simulink model "stereo_ibvs_core"  (R2025b)
settings: Solver=FixedStepDiscrete  StartTime=0.0  StopTime=inf  FixedStep=cfg.Ts  RelTol=1e-3
InitFcn:
  | modelFile__ = get_param(bdroot,'FileName'); modelDir__ = fileparts(modelFile__); config1__ = fullfile(modelDir__,'stereo_ibvs_config.m'); config2__ = fullfile(fileparts(modelDir__),'config','stereo_ibvs_config.m'); if isfile(config1__), run(config1__); elseif isfile(config2__), run(config2__); else, error('StereoIBVS:ConfigNotFound','找不到stereo_ibvs_config.m。'); end; clear modelFile__ modelDir__ config1__ config2__;
undefined symbols (not defined in the file or in its folder): cfg
libraries: robotmaniplib x2
settings Model: Creator=harry  LastModifiedBy=hlc

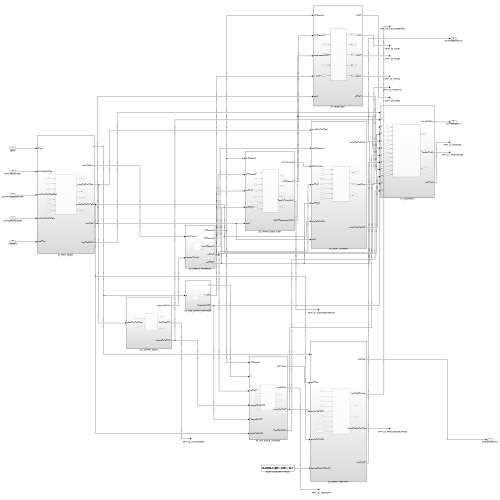
[thumbnail: Simulink's stored preview of the top-level diagram]
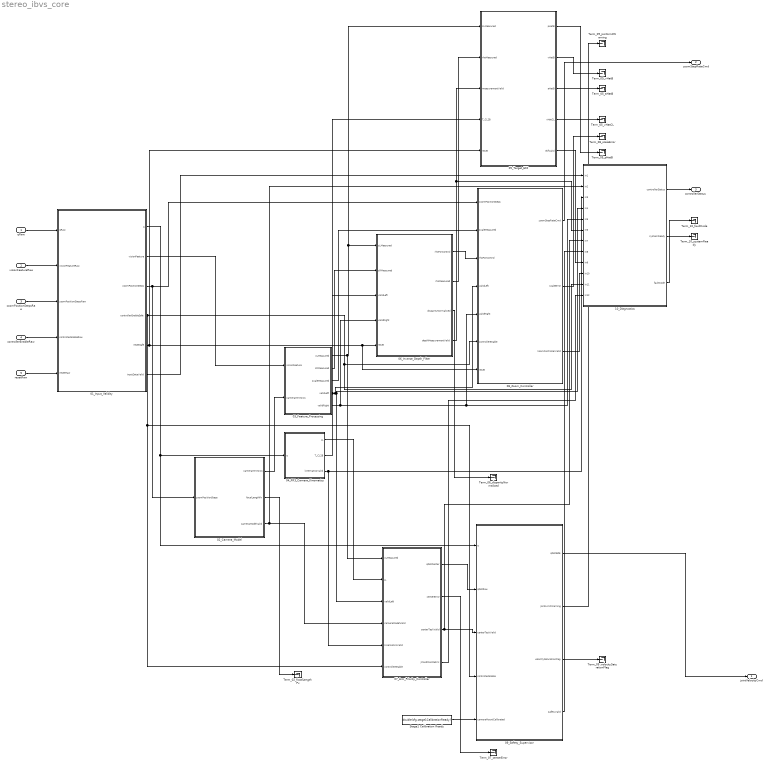
== system stereo_ibvs_core ==
  qRaw : Inport  OutDataTypeStr=double  PortDimensions=[7 1]
  visionFeatureRaw : Inport  Port=2  PortDimensions=[8 1]
  zoomPositionStepsRaw : Inport  Port=3  PortDimensions=[2 1]
  controllerEnableRaw : Inport  Port=4  OutDataTypeStr=double  PortDimensions=1
  resetRaw : Inport  Port=5  OutDataTypeStr=double  PortDimensions=1
  01_Input_Validity : Subsystem
  02_Camera_Model : Subsystem
  03_Feature_Processing : Subsystem  Description=将像素坐标转换为左右相机归一化坐标，并检查输入有效性。
  04_FR3_Camera_Kinematics : Subsystem
  05_Target_EKF : Subsystem
  06_Inverse_Depth_Filter : Subsystem
  07_Arm_Priority_Controller : Subsystem
  08_Zoom_Controller : Subsystem
  09_Safety_Supervisor : Subsystem
  10_Diagnostics : Subsystem
  Stage1 Calibration Ready : Constant  Value=double(cfg.stage1CalibrationReady)  SampleTime=-1
  Term_02_focalLengthPx : Terminator
  Term_05_aHatB : Terminator
  Term_05_pHatB : Terminator
  Term_05_vHatB : Terminator
  Term_05_vHatCL : Terminator
  Term_06_disparityNormalized : Terminator
  Term_07_centerError : Terminator
  Term_08_scaleError : Terminator
  Term_09_jointLimitWarning : Terminator
  Term_09_velocitySaturationFlag : Terminator
  Term_10_faultCode : Terminator
  Term_10_systemReady : Terminator
  jointVelocityCmd : Outport  PortDimensions=[7 1]
  zoomStepRateCmd : Outport  Port=2  PortDimensions=[2 1]
  controllerStatus : Outport  Port=3  PortDimensions=[12 1]
  wires:
  10_Diagnostics/3(faultCode) -> Term_10_faultCode/1
  10_Diagnostics/1(controllerStatus) -> controllerStatus/1
  09_Safety_Supervisor/4(safetyValid) -> 10_Diagnostics/8(In8)
  09_Safety_Supervisor/1(qDotSafe) -> jointVelocityCmd/1
  08_Zoom_Controller/2(scaleError) -> Term_08_scaleError/1
  05_Target_EKF/3(aHatB) -> Term_05_aHatB/1
  Stage1 Calibration Ready/1 -> 09_Safety_Supervisor/5(cameraMountCalibrated)
  08_Zoom_Controller/3(zoomControllerValid) -> 10_Diagnostics/10(In10)
  07_Arm_Priority_Controller/4(jConditionMetric) -> 10_Diagnostics/12(In12)
  01_Input_Validity/6(inputDataValid) -> 10_Diagnostics/1(In1)
  01_Input_Validity/5(resetSafe) -> 06_Inverse_Depth_Filter/5(reset), 08_Zoom_Controller/7(reset), 05_Target_EKF/5(reset)
  01_Input_Validity/2(visionFeature) -> 03_Feature_Processing/1(visionFeature)
  01_Input_Validity/1(q) -> 09_Safety_Supervisor/1(q), 04_FR3_Camera_Kinematics/1(q)
  02_Camera_Model/1(cameraIntrinsics) -> 03_Feature_Processing/2(cameraIntrinsics)
  02_Camera_Model/2(focalLengthPx) -> Term_02_focalLengthPx/1
  08_Zoom_Controller/1(zoomStepRateCmd) -> zoomStepRateCmd/1
  03_Feature_Processing/3(scaleMeasured) -> 08_Zoom_Controller/2(scaleMeasured)
  05_Target_EKF/4(vHatCL) -> Term_05_vHatCL/1
  resetRaw/1 -> 01_Input_Validity/5(resetRaw)
  controllerEnableRaw/1 -> 01_Input_Validity/4(controllerEnableRaw)
  07_Arm_Priority_Controller/1(qDotCenter) -> 09_Safety_Supervisor/2(qDotRaw)
  09_Safety_Supervisor/2(jointLimitWarning) -> Term_09_jointLimitWarning/1
  05_Target_EKF/5(ekfValid) -> 10_Diagnostics/9(In9)
  05_Target_EKF/1(pHatB) -> Term_05_pHatB/1
  zoomPositionStepsRaw/1 -> 01_Input_Validity/3(zoomPositionStepsRaw)
  visionFeatureRaw/1 -> 01_Input_Validity/2(visionFeatureRaw)
  06_Inverse_Depth_Filter/4(depthMeasurementValid) -> 05_Target_EKF/3(measurementValid), 10_Diagnostics/6(In6)
  01_Input_Validity/4(controllerEnableSafe) -> 09_Safety_Supervisor/4(controllerEnable), 07_Arm_Priority_Controller/6(controllerEnable), 08_Zoom_Controller/6(controllerEnable), 10_Diagnostics/11(In11)
  qRaw/1 -> 01_Input_Validity/1(qRaw)
  03_Feature_Processing/1(cLMeasured) -> 06_Inverse_Depth_Filter/1(cLMeasured), 05_Target_EKF/1(cLMeasured), 07_Arm_Priority_Controller/1(cLMeasured)
  03_Feature_Processing/4(validLeft) -> 07_Arm_Priority_Controller/3(validLeft), 10_Diagnostics/4(In4), 08_Zoom_Controller/4(validLeft), 06_Inverse_Depth_Filter/3(validLeft)
  03_Feature_Processing/5(validRight) -> 08_Zoom_Controller/5(validRight), 10_Diagnostics/5(In5), 06_Inverse_Depth_Filter/4(validRight)
  10_Diagnostics/2(systemReady) -> Term_10_systemReady/1
  02_Camera_Model/3(cameraModelValid) -> 10_Diagnostics/2(In2), 07_Arm_Priority_Controller/4(cameraModelValid)
  04_FR3_Camera_Kinematics/3(kinematicsValid) -> 07_Arm_Priority_Controller/5(kinematicsValid), 10_Diagnostics/3(In3)
  05_Target_EKF/2(vHatB) -> Term_05_vHatB/1
  07_Arm_Priority_Controller/3(centerTaskValid) -> 09_Safety_Supervisor/3(centerTaskValid), 10_Diagnostics/7(In7)
  09_Safety_Supervisor/3(velocitySaturationFlag) -> Term_09_velocitySaturationFlag/1
  04_FR3_Camera_Kinematics/2(T_CL2B) -> 05_Target_EKF/4(T_CL2B)
  03_Feature_Processing/2(cRMeasured) -> 06_Inverse_Depth_Filter/2(cRMeasured)
  06_Inverse_Depth_Filter/2(rhoMeasured) -> 05_Target_EKF/2(rhoMeasured)
  01_Input_Validity/3(zoomPositionSteps) -> 02_Camera_Model/1(zoomPositionSteps), 08_Zoom_Controller/1(zoomPositionSteps)
  07_Arm_Priority_Controller/2(centerError) -> Term_07_centerError/1
  06_Inverse_Depth_Filter/1(rhoForControl) -> 08_Zoom_Controller/3(rhoForControl)
  04_FR3_Camera_Kinematics/1(JL) -> 07_Arm_Priority_Controller/2(JL)
  06_Inverse_Depth_Filter/3(disparityNormalized) -> Term_06_disparityNormalized/1

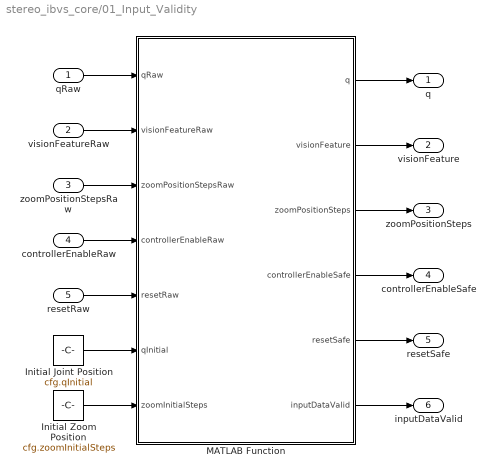
== system stereo_ibvs_core/01_Input_Validity ==
  qRaw : Inport  PortDimensions=[7 1]
  visionFeatureRaw : Inport  Port=2  PortDimensions=[8 1]
  zoomPositionStepsRaw : Inport  Port=3  PortDimensions=[2 1]
  controllerEnableRaw : Inport  Port=4  PortDimensions=1
  resetRaw : Inport  Port=5  PortDimensions=1
  Initial Joint Position : Constant  Value=cfg.qInitial  VectorParams1D=off
  Initial Zoom Position : Constant  Value=cfg.zoomInitialSteps  VectorParams1D=off
  MATLAB Function : MATLAB Function  TreatAsAtomicUnit=on
  q : Outport  PortDimensions=[7 1]
  visionFeature : Outport  Port=2  PortDimensions=[8 1]
  zoomPositionSteps : Outport  Port=3  PortDimensions=[2 1]
  controllerEnableSafe : Outport  Port=4  PortDimensions=1
  resetSafe : Outport  Port=5  PortDimensions=1
  inputDataValid : Outport  Port=6  PortDimensions=1
  wires:
  MATLAB Function/1(q) -> q/1
  MATLAB Function/2(visionFeature) -> visionFeature/1
  MATLAB Function/3(zoomPositionSteps) -> zoomPositionSteps/1
  MATLAB Function/4(controllerEnableSafe) -> controllerEnableSafe/1
  MATLAB Function/5(resetSafe) -> resetSafe/1
  MATLAB Function/6(inputDataValid) -> inputDataValid/1
  qRaw/1 -> MATLAB Function/1(qRaw)
  visionFeatureRaw/1 -> MATLAB Function/2(visionFeatureRaw)
  zoomPositionStepsRaw/1 -> MATLAB Function/3(zoomPositionStepsRaw)
  controllerEnableRaw/1 -> MATLAB Function/4(controllerEnableRaw)
  resetRaw/1 -> MATLAB Function/5(resetRaw)
  Initial Joint Position/1 -> MATLAB Function/6(qInitial)
  Initial Zoom Position/1 -> MATLAB Function/7(zoomInitialSteps)

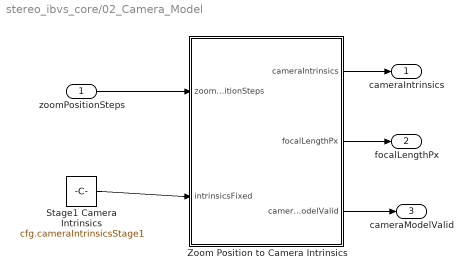
== system stereo_ibvs_core/02_Camera_Model ==
  zoomPositionSteps : Inport  PortDimensions=[2 1]
  Stage1 Camera Intrinsics : Constant  Value=cfg.cameraIntrinsicsStage1  VectorParams1D=off
  Zoom Position to Camera Intrinsics : MATLAB Function  TreatAsAtomicUnit=on
  cameraIntrinsics : Outport  PortDimensions=[8 1]
  focalLengthPx : Outport  Port=2  PortDimensions=[2 1]
  cameraModelValid : Outport  Port=3  PortDimensions=1
  wires:
  zoomPositionSteps/1 -> Zoom Position to Camera Intrinsics/1(zoomPositionSteps)
  Stage1 Camera Intrinsics/1 -> Zoom Position to Camera Intrinsics/2(intrinsicsFixed)
  Zoom Position to Camera Intrinsics/3(cameraModelValid) -> cameraModelValid/1
  Zoom Position to Camera Intrinsics/2(focalLengthPx) -> focalLengthPx/1
  Zoom Position to Camera Intrinsics/1(cameraIntrinsics) -> cameraIntrinsics/1

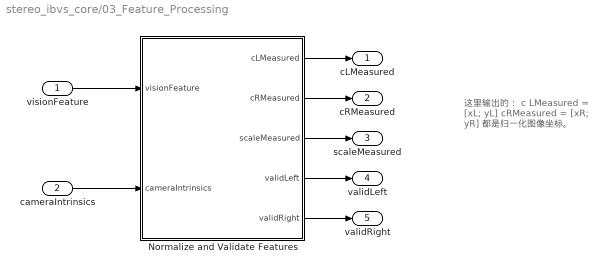
== system stereo_ibvs_core/03_Feature_Processing ==
  note: 这里输出的：
      | c LMeasured = [xL; yL]
      | cRMeasured = [xR; yR]
      | 都是归一化图像坐标。
  visionFeature : Inport  PortDimensions=[8 1]
  cameraIntrinsics : Inport  Description=|  Port=2  PortDimensions=[8 1]
      | 顺序固定为：
      | [fxL; fyL; cxL; cyL; fxR; fyR; cxR; cyR]
  Normalize and Validate Features : MATLAB Function  TreatAsAtomicUnit=on
  cLMeasured : Outport  PortDimensions=[2 1]
  cRMeasured : Outport  Port=2  PortDimensions=[2 1]
  scaleMeasured : Outport  Port=3  PortDimensions=[2 1]
  validLeft : Outport  Port=4  PortDimensions=1
  validRight : Outport  Port=5  PortDimensions=1
  wires:
  cameraIntrinsics/1 -> Normalize and Validate Features/2(cameraIntrinsics)
  visionFeature/1 -> Normalize and Validate Features/1(visionFeature)
  Normalize and Validate Features/2(cRMeasured) -> cRMeasured/1
  Normalize and Validate Features/4(validLeft) -> validLeft/1
  Normalize and Validate Features/5(validRight) -> validRight/1
  Normalize and Validate Features/3(scaleMeasured) -> scaleMeasured/1
  Normalize and Validate Features/1(cLMeasured) -> cLMeasured/1

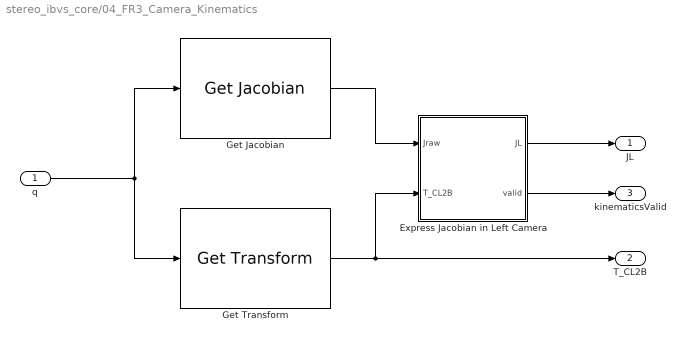
== system stereo_ibvs_core/04_FR3_Camera_Kinematics ==
  q : Inport  PortDimensions=[7 1]
  Express Jacobian in Left Camera : MATLAB Function  TreatAsAtomicUnit=on
  Get Jacobian : robotmaniplib/Get Jacobian  Description=关节速度如何产生左相机光心的运动速度。该速度默认在 base 坐标系表达  RigidBodyTree=cfg.robot  EndEffector=left_camera_optical  SimulateUsing=Interpreted execution
  Get Transform : robotmaniplib/Get Transform  Description=它把左相机坐标系(source)中的点转换到 base 坐标系(target)  RigidBodyTree=cfg.robot  SourceBody=left_camera_optical  TargetBody=base  SimulateUsing=Interpreted execution
  JL : Outport  PortDimensions=[6 7]
  T_CL2B : Outport  Port=2  PortDimensions=[4 4]
  kinematicsValid : Outport  Port=3  PortDimensions=1
  wires:
  q/1 -> Get Jacobian/1, Get Transform/1
  Get Jacobian/1 -> Express Jacobian in Left Camera/1(Jraw)
  Get Transform/1 -> T_CL2B/1, Express Jacobian in Left Camera/2(T_CL2B)
  Express Jacobian in Left Camera/1(JL) -> JL/1
  Express Jacobian in Left Camera/2(valid) -> kinematicsValid/1

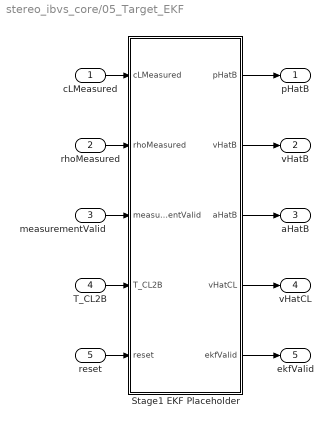
== system stereo_ibvs_core/05_Target_EKF ==
  cLMeasured : Inport  PortDimensions=[2 1]
  rhoMeasured : Inport  Port=2  PortDimensions=1
  measurementValid : Inport  Port=3  PortDimensions=1
  T_CL2B : Inport  Port=4  PortDimensions=[4 4]
  reset : Inport  Port=5  PortDimensions=1
  Stage1 EKF Placeholder : MATLAB Function  TreatAsAtomicUnit=on
  pHatB : Outport  PortDimensions=[3 1]
  vHatB : Outport  Port=2  PortDimensions=[3 1]
  aHatB : Outport  Port=3  PortDimensions=[3 1]
  vHatCL : Outport  Port=4  PortDimensions=[3 1]
  ekfValid : Outport  Port=5  PortDimensions=1
  wires:
  cLMeasured/1 -> Stage1 EKF Placeholder/1(cLMeasured)
  rhoMeasured/1 -> Stage1 EKF Placeholder/2(rhoMeasured)
  measurementValid/1 -> Stage1 EKF Placeholder/3(measurementValid)
  T_CL2B/1 -> Stage1 EKF Placeholder/4(T_CL2B)
  reset/1 -> Stage1 EKF Placeholder/5(reset)
  Stage1 EKF Placeholder/1(pHatB) -> pHatB/1
  Stage1 EKF Placeholder/2(vHatB) -> vHatB/1
  Stage1 EKF Placeholder/3(aHatB) -> aHatB/1
  Stage1 EKF Placeholder/4(vHatCL) -> vHatCL/1
  Stage1 EKF Placeholder/5(ekfValid) -> ekfValid/1

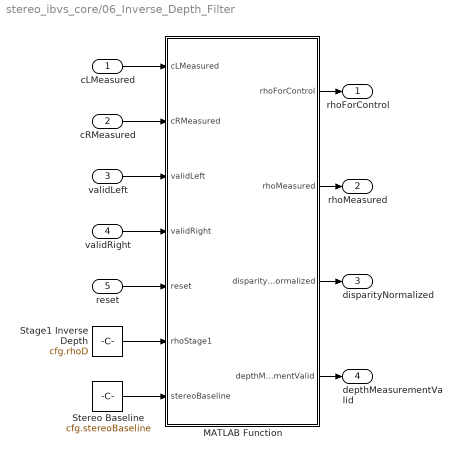
== system stereo_ibvs_core/06_Inverse_Depth_Filter ==
  cLMeasured : Inport  PortDimensions=[2 1]
  cRMeasured : Inport  Port=2  PortDimensions=[2 1]
  validLeft : Inport  Port=3  PortDimensions=1
  validRight : Inport  Port=4  PortDimensions=1
  reset : Inport  Port=5  PortDimensions=1
  MATLAB Function : MATLAB Function  TreatAsAtomicUnit=on
  Stage1 Inverse Depth : Constant  Value=cfg.rhoD  VectorParams1D=off
  Stereo Baseline : Constant  Value=cfg.stereoBaseline  VectorParams1D=off
  rhoForControl : Outport  PortDimensions=1
  rhoMeasured : Outport  Port=2  PortDimensions=1
  disparityNormalized : Outport  Port=3  PortDimensions=1
  depthMeasurementValid : Outport  Port=4  PortDimensions=1
  wires:
  cLMeasured/1 -> MATLAB Function/1(cLMeasured)
  cRMeasured/1 -> MATLAB Function/2(cRMeasured)
  validLeft/1 -> MATLAB Function/3(validLeft)
  validRight/1 -> MATLAB Function/4(validRight)
  reset/1 -> MATLAB Function/5(reset)
  Stage1 Inverse Depth/1 -> MATLAB Function/6(rhoStage1)
  Stereo Baseline/1 -> MATLAB Function/7(stereoBaseline)
  MATLAB Function/1(rhoForControl) -> rhoForControl/1
  MATLAB Function/2(rhoMeasured) -> rhoMeasured/1
  MATLAB Function/3(disparityNormalized) -> disparityNormalized/1
  MATLAB Function/4(depthMeasurementValid) -> depthMeasurementValid/1

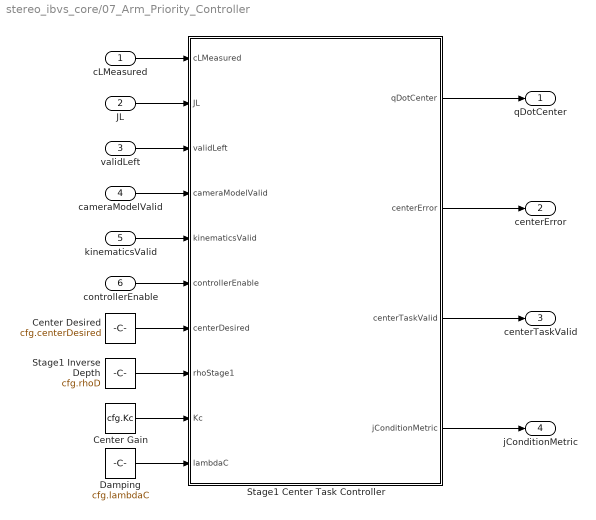
== system stereo_ibvs_core/07_Arm_Priority_Controller ==
  cLMeasured : Inport  PortDimensions=[2 1]
  JL : Inport  Port=2  PortDimensions=[6 7]
  validLeft : Inport  Port=3  PortDimensions=1
  cameraModelValid : Inport  Port=4  PortDimensions=1
  kinematicsValid : Inport  Port=5  PortDimensions=1
  controllerEnable : Inport  Port=6  PortDimensions=1
  Center Desired : Constant  Value=cfg.centerDesired  VectorParams1D=off
  Center Gain : Constant  Value=cfg.Kc  VectorParams1D=off
  Damping : Constant  Value=cfg.lambdaC  VectorParams1D=off
  Stage1 Center Task Controller : MATLAB Function  TreatAsAtomicUnit=on
  Stage1 Inverse Depth : Constant  Value=cfg.rhoD  VectorParams1D=off
  qDotCenter : Outport  PortDimensions=[7 1]
  centerError : Outport  Port=2  PortDimensions=[2 1]
  centerTaskValid : Outport  Port=3  PortDimensions=1
  jConditionMetric : Outport  Port=4  PortDimensions=1
  wires:
  kinematicsValid/1 -> Stage1 Center Task Controller/5(kinematicsValid)
  cameraModelValid/1 -> Stage1 Center Task Controller/4(cameraModelValid)
  JL/1 -> Stage1 Center Task Controller/2(JL)
  cLMeasured/1 -> Stage1 Center Task Controller/1(cLMeasured)
  validLeft/1 -> Stage1 Center Task Controller/3(validLeft)
  controllerEnable/1 -> Stage1 Center Task Controller/6(controllerEnable)
  Center Desired/1 -> Stage1 Center Task Controller/7(centerDesired)
  Stage1 Inverse Depth/1 -> Stage1 Center Task Controller/8(rhoStage1)
  Center Gain/1 -> Stage1 Center Task Controller/9(Kc)
  Damping/1 -> Stage1 Center Task Controller/10(lambdaC)
  Stage1 Center Task Controller/4(jConditionMetric) -> jConditionMetric/1
  Stage1 Center Task Controller/3(centerTaskValid) -> centerTaskValid/1
  Stage1 Center Task Controller/2(centerError) -> centerError/1
  Stage1 Center Task Controller/1(qDotCenter) -> qDotCenter/1

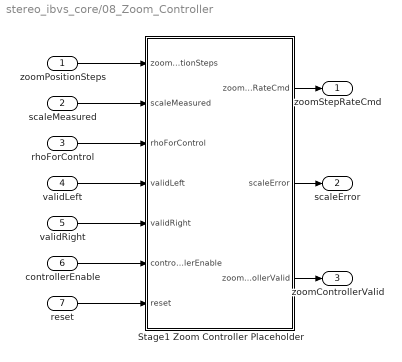
== system stereo_ibvs_core/08_Zoom_Controller ==
  zoomPositionSteps : Inport  PortDimensions=[2 1]
  scaleMeasured : Inport  Port=2  PortDimensions=[2 1]
  rhoForControl : Inport  Port=3  PortDimensions=1
  validLeft : Inport  Port=4  PortDimensions=1
  validRight : Inport  Port=5  PortDimensions=1
  controllerEnable : Inport  Port=6  PortDimensions=1
  reset : Inport  Port=7  PortDimensions=1
  Stage1 Zoom Controller Placeholder : MATLAB Function  TreatAsAtomicUnit=on
  zoomStepRateCmd : Outport  PortDimensions=[2 1]
  scaleError : Outport  Port=2  PortDimensions=[2 1]
  zoomControllerValid : Outport  Port=3  PortDimensions=1
  wires:
  Stage1 Zoom Controller Placeholder/1(zoomStepRateCmd) -> zoomStepRateCmd/1
  Stage1 Zoom Controller Placeholder/2(scaleError) -> scaleError/1
  Stage1 Zoom Controller Placeholder/3(zoomControllerValid) -> zoomControllerValid/1
  zoomPositionSteps/1 -> Stage1 Zoom Controller Placeholder/1(zoomPositionSteps)
  scaleMeasured/1 -> Stage1 Zoom Controller Placeholder/2(scaleMeasured)
  rhoForControl/1 -> Stage1 Zoom Controller Placeholder/3(rhoForControl)
  validLeft/1 -> Stage1 Zoom Controller Placeholder/4(validLeft)
  validRight/1 -> Stage1 Zoom Controller Placeholder/5(validRight)
  controllerEnable/1 -> Stage1 Zoom Controller Placeholder/6(controllerEnable)
  reset/1 -> Stage1 Zoom Controller Placeholder/7(reset)

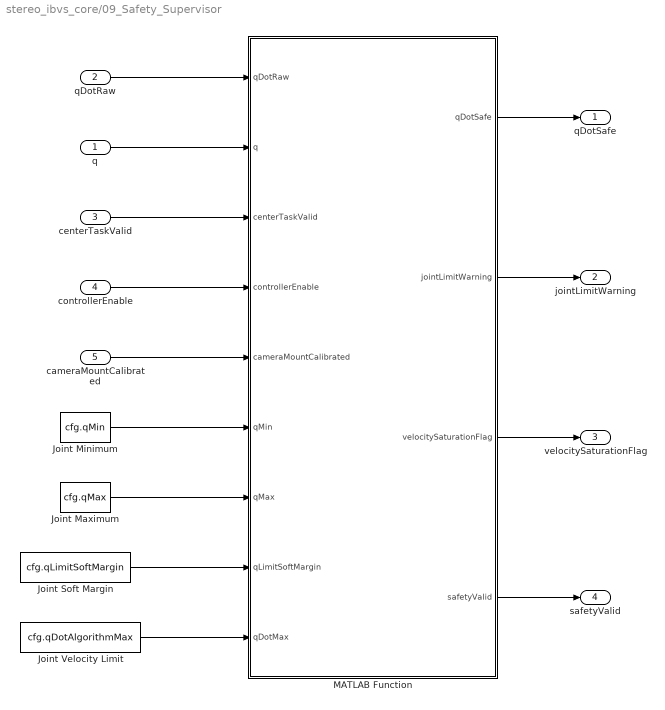
== system stereo_ibvs_core/09_Safety_Supervisor ==
  q : Inport  PortDimensions=[7 1]
  qDotRaw : Inport  Port=2  PortDimensions=[7 1]
  centerTaskValid : Inport  Port=3  PortDimensions=1
  controllerEnable : Inport  Port=4  PortDimensions=1
  cameraMountCalibrated : Inport  Port=5  PortDimensions=1
  Joint Maximum : Constant  Value=cfg.qMax  VectorParams1D=off
  Joint Minimum : Constant  Value=cfg.qMin  VectorParams1D=off
  Joint Soft Margin : Constant  Value=cfg.qLimitSoftMargin  VectorParams1D=off
  Joint Velocity Limit : Constant  Value=cfg.qDotAlgorithmMax  VectorParams1D=off
  MATLAB Function : MATLAB Function  TreatAsAtomicUnit=on
  qDotSafe : Outport  PortDimensions=[7 1]
  jointLimitWarning : Outport  Port=2  PortDimensions=[7 1]
  velocitySaturationFlag : Outport  Port=3  PortDimensions=[7 1]
  safetyValid : Outport  Port=4  PortDimensions=1
  wires:
  MATLAB Function/2(jointLimitWarning) -> jointLimitWarning/1
  MATLAB Function/3(velocitySaturationFlag) -> velocitySaturationFlag/1
  MATLAB Function/1(qDotSafe) -> qDotSafe/1
  Joint Velocity Limit/1 -> MATLAB Function/9(qDotMax)
  MATLAB Function/4(safetyValid) -> safetyValid/1
  Joint Maximum/1 -> MATLAB Function/7(qMax)
  Joint Minimum/1 -> MATLAB Function/6(qMin)
  controllerEnable/1 -> MATLAB Function/4(controllerEnable)
  Joint Soft Margin/1 -> MATLAB Function/8(qLimitSoftMargin)
  centerTaskValid/1 -> MATLAB Function/3(centerTaskValid)
  cameraMountCalibrated/1 -> MATLAB Function/5(cameraMountCalibrated)
  q/1 -> MATLAB Function/2(q)
  qDotRaw/1 -> MATLAB Function/1(qDotRaw)

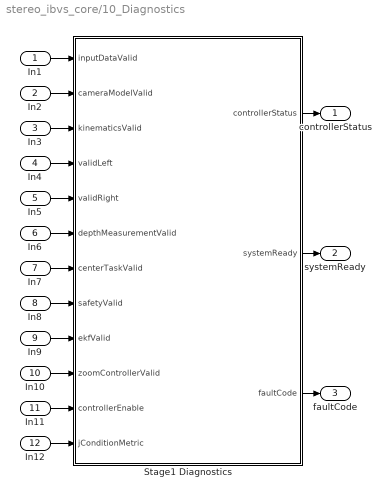
== system stereo_ibvs_core/10_Diagnostics ==
  In1 : Inport  PortDimensions=1
  In2 : Inport  Port=2  PortDimensions=1
  In3 : Inport  Port=3  PortDimensions=1
  In4 : Inport  Port=4  PortDimensions=1
  In5 : Inport  Port=5  PortDimensions=1
  In6 : Inport  Port=6  PortDimensions=1
  In7 : Inport  Port=7  PortDimensions=1
  In8 : Inport  Port=8  PortDimensions=1
  In9 : Inport  Port=9  PortDimensions=1
  In10 : Inport  Port=10  PortDimensions=1
  In11 : Inport  Port=11  PortDimensions=1
  In12 : Inport  Port=12  PortDimensions=1
  Stage1 Diagnostics : MATLAB Function  TreatAsAtomicUnit=on
  controllerStatus : Outport  PortDimensions=[12 1]
  systemReady : Outport  Port=2  PortDimensions=1
  faultCode : Outport  Port=3  PortDimensions=1
  wires:
  In1/1 -> Stage1 Diagnostics/1(inputDataValid)
  In2/1 -> Stage1 Diagnostics/2(cameraModelValid)
  In3/1 -> Stage1 Diagnostics/3(kinematicsValid)
  In4/1 -> Stage1 Diagnostics/4(validLeft)
  In5/1 -> Stage1 Diagnostics/5(validRight)
  In6/1 -> Stage1 Diagnostics/6(depthMeasurementValid)
  In7/1 -> Stage1 Diagnostics/7(centerTaskValid)
  In8/1 -> Stage1 Diagnostics/8(safetyValid)
  In9/1 -> Stage1 Diagnostics/9(ekfValid)
  In10/1 -> Stage1 Diagnostics/10(zoomControllerValid)
  In11/1 -> Stage1 Diagnostics/11(controllerEnable)
  In12/1 -> Stage1 Diagnostics/12(jConditionMetric)
  Stage1 Diagnostics/1(controllerStatus) -> controllerStatus/1
  Stage1 Diagnostics/2(systemReady) -> systemReady/1
  Stage1 Diagnostics/3(faultCode) -> faultCode/1

== matlab function stereo_ibvs_core/06_Inverse_Depth_Filter/MATLAB Function ==
  data: cLMeasured input; rhoForControl output; cRMeasured input; validLeft input; validRight input; reset input; rhoStage1 input; stereoBaseline input; rhoMeasured output; disparityNormalized output; depthMeasurementValid output
function [rhoForControl,rhoMeasured,disparityNormalized, ...
    depthMeasurementValid] = ...
    fcn(cLMeasured,cRMeasured,validLeft,validRight,reset, ...
    rhoStage1,stereoBaseline)
%#codegen
% 代码作用：
% 为控制器提供目标逆深度。
% Stage 1暂时使用固定逆深度rhoStage1。
% 同时计算双目归一化视差和逆深度测量值，仅用于诊断。
% Stage 2将在此处加入真正的逆深度预测和校正滤波。

% 输入参数含义：
% cLMeasured：
% 左相机归一化目标坐标，[xL; yL]。
%
% cRMeasured：
% 右相机归一化目标坐标，[xR; yR]。
%
% validLeft、validRight：
% 左右相机目标检测是否有效。
%
% reset：
% 估计器复位信号。
%
% rhoStage1：
% Stage 1使用的固定逆深度，rho=1/Z，单位1/m。
%
% stereoBaseline：
% 左右相机光心基线长度，单位m。

% 输出参数含义：
% rhoForControl：
% 提供给机械臂控制器使用的逆深度，单位1/m。
%
% rhoMeasured：
% 根据双目归一化视差计算的逆深度测量值，单位1/m。
%
% disparityNormalized：
% 左右相机水平方向归一化视差，xL-xR。
%
% depthMeasurementValid：
% 当前双目逆深度测量是否有效，有效为1，无效为0。

rhoForControl = 0;
rhoMeasured = 0;
disparityNormalized = 0;
depthMeasurementValid = 0;

cL = reshape(cLMeasured,2,1);
cR = reshape(cRMeasured,2,1);

% 检查输入是否合法。
if any(~isfinite(cL)) || ...
        any(~isfinite(cR)) || ...
        ~isfinite(rhoStage1) || ...
        ~isfinite(stereoBaseline)
    return;
end

if rhoStage1 <= 0
    return;
end

% Stage 1始终使用固定逆深度。
rhoForControl = rhoStage1;

% 复位时不使用双目测量。
if reset > 0.5
    return;
end

% 只有左右目标均有效且基线大于零时才计算双目测量。
if validLeft <= 0.5 || ...
        validRight <= 0.5 || ...
        stereoBaseline <= 0
    return;
end

disparityNormalized = cL(1) - cR(1);

rhoCandidate = ...
    disparityNormalized / stereoBaseline;

% 逆深度必须为正数。
if isfinite(rhoCandidate) && rhoCandidate > 0
    rhoMeasured = rhoCandidate;
    depthMeasurementValid = 1;
end
end

== matlab function stereo_ibvs_core/05_Target_EKF/Stage1 EKF Placeholder ==
  data: cLMeasured input; pHatB output; rhoMeasured input; measurementValid input; T_CL2B input; reset input; vHatB output; aHatB output; vHatCL output; ekfValid output
function [pHatB,vHatB,aHatB,vHatCL,ekfValid] = ...
    fcn(cLMeasured,rhoMeasured,measurementValid,T_CL2B,reset)
%#codegen
% 代码作用：
% 本函数是Stage 1的目标运动EKF占位模块。
% Stage 1不估计目标位置、速度和加速度，因此所有估计量输出为零，
% ekfValid输出为0。
% Stage 4将在保持输入输出接口不变的前提下，替换为正式的九状态EKF。

% 输入参数含义：
% cLMeasured：
% 左相机中的目标归一化坐标，格式为[xL; yL]。
%
% rhoMeasured：
% 双目测量得到的目标逆深度，单位为1/m。
%
% measurementValid：
% 当前视觉位置和逆深度测量是否有效。
%
% T_CL2B：
% 左相机坐标系到机械臂基座坐标系的齐次变换矩阵。
%
% reset：
% EKF复位信号，复位时为1。

% 输出参数含义：
% pHatB：
% 目标在机械臂基座坐标系中的估计位置，单位为m。
%
% vHatB：
% 目标在机械臂基座坐标系中的估计速度，单位为m/s。
%
% aHatB：
% 目标在机械臂基座坐标系中的估计加速度，单位为m/s^2。
%
% vHatCL：
% 目标速度在左相机坐标系中的表达，单位为m/s。
%
% ekfValid：
% EKF估计结果是否可以用于控制，有效为1，无效为0。

pHatB = zeros(3,1);
vHatB = zeros(3,1);
aHatB = zeros(3,1);
vHatCL = zeros(3,1);
ekfValid = 0;

% Stage 1不使用这些输入。
% 下面的有限值检查用于提前固定各端口的数据尺寸和类型。
cL = reshape(cLMeasured,2,1);
T = reshape(T_CL2B,4,4);

inputsFinite = ...
    all(isfinite(cL)) && ...
    isfinite(rhoMeasured) && ...
    isfinite(measurementValid) && ...
    all(isfinite(T(:))) && ...
    isfinite(reset);

if ~inputsFinite
    return;
end

% Stage 1明确禁止启用目标运动前馈。
ekfValid = 0;
end

== matlab function stereo_ibvs_core/08_Zoom_Controller/Stage1 Zoom Controller Placeholder ==
  data: zoomPositionSteps input; zoomStepRateCmd output; scaleMeasured input; rhoForControl input; validLeft input; validRight input; controllerEnable input; reset input; scaleError output; zoomControllerValid output
function [zoomStepRateCmd,scaleError,zoomControllerValid] = ...
    fcn(zoomPositionSteps,scaleMeasured,rhoForControl, ...
    validLeft,validRight,controllerEnable,reset)
%#codegen
% 代码作用：
% 本函数是Stage 1的变焦控制器占位模块。
% Stage 1不控制左右变焦电机，因此始终输出零步进速度。
% Stage 5将在保持输入输出接口基本不变的情况下，
% 加入尺度误差控制和步进电机位置到焦距的标定模型。

% 输入参数含义：
% zoomPositionSteps：
% 左右变焦步进电机当前累计位置，
% 格式为[leftSteps; rightSteps]。
%
% scaleMeasured：
% 左右相机检测到的目标尺度，
% 格式为[scaleL; scaleR]。
%
% rhoForControl：
% 当前控制使用的目标逆深度，单位为1/m。
%
% validLeft、validRight：
% 左右相机目标检测是否有效。
%
% controllerEnable：
% 控制器总使能信号。
%
% reset：
% 变焦控制器复位信号。

% 输出参数含义：
% zoomStepRateCmd：
% 左右步进电机目标速度，
% 格式为[leftStepRate; rightStepRate]，单位为steps/s。
%
% scaleError：
% 左右相机目标尺度误差。
% Stage 1未设置尺度控制目标，因此暂时输出零。
%
% zoomControllerValid：
% 变焦控制器输出是否有效。
% Stage 1未启用变焦控制，因此始终输出0。

zoomStepRateCmd = zeros(2,1);
scaleError = zeros(2,1);
zoomControllerValid = 0;

steps = reshape(zoomPositionSteps,2,1);
scale = reshape(scaleMeasured,2,1);

% 检查输入数据是否为有限值，固定端口尺寸和类型。
inputsFinite = ...
    all(isfinite(steps)) && ...
    all(isfinite(scale)) && ...
    isfinite(rhoForControl) && ...
    isfinite(validLeft) && ...
    isfinite(validRight) && ...
    isfinite(controllerEnable) && ...
    isfinite(reset);

if ~inputsFinite
    return;
end

% Stage 1明确禁止变焦电机运动。
zoomStepRateCmd = zeros(2,1);
scaleError = zeros(2,1);
zoomControllerValid = 0;
end

== matlab function stereo_ibvs_core/10_Diagnostics/Stage1 Diagnostics ==
  data: inputDataValid input; controllerStatus output; cameraModelValid input; kinematicsValid input; validLeft input; validRight input; depthMeasurementValid input; centerTaskValid input; safetyValid input; ekfValid input; zoomControllerValid input; controllerEnable input; jConditionMetric input; systemReady output; faultCode output
function [controllerStatus,systemReady,faultCode] = ...
    fcn(inputDataValid,cameraModelValid,kinematicsValid, ...
    validLeft,validRight,depthMeasurementValid, ...
    centerTaskValid,safetyValid,ekfValid,zoomControllerValid, ...
    controllerEnable,jConditionMetric)
%#codegen
% 代码作用：
% 汇总Stage 1各子系统的有效状态，判断当前控制链路是否准备完成，
% 并输出统一的状态向量和故障代码，便于后续记录和ROS监控。

% 输入参数含义：
% inputDataValid：
% 顶层输入数据是否有效。
%
% cameraModelValid：
% 相机内参模型是否有效。
%
% kinematicsValid：
% FR3运动学和左相机雅可比是否有效。
%
% validLeft、validRight：
% 左右相机目标检测是否有效。
%
% depthMeasurementValid：
% 双目逆深度测量是否有效。
%
% centerTaskValid：
% 左相机中心任务计算是否有效。
%
% safetyValid：
% 安全模块是否允许输出关节速度。
%
% ekfValid：
% 目标运动EKF是否有效。
% Stage 1中固定为0。
%
% zoomControllerValid：
% 变焦控制器是否有效。
% Stage 1中固定为0。
%
% controllerEnable：
% 控制器总使能信号。
%
% jConditionMetric：
% 中心任务雅可比条件指标。

% 输出参数含义：
% controllerStatus：
% 统一状态向量，格式为：
% [inputDataValid;
%  cameraModelValid;
%  kinematicsValid;
%  validLeft;
%  validRight;
%  depthMeasurementValid;
%  centerTaskValid;
%  safetyValid;
%  ekfValid;
%  zoomControllerValid;
%  controllerEnable;
%  jConditionMetric]
%
% systemReady：
% Stage 1中心控制链路是否准备完成。
% 准备完成为1，否则为0。
%
% faultCode：
% 当前主要故障代码：
% 0：无故障
% 1：输入数据无效
% 2：相机模型无效
% 3：机械臂运动学无效
% 4：左相机目标无效
% 5：中心任务计算无效
% 6：安全模块未通过
% 7：控制器未使能

controllerStatus = zeros(12,1);
systemReady = 0;
faultCode = 0;

statusInputs = [
    inputDataValid
    cameraModelValid
    kinematicsValid
    validLeft
    validRight
    depthMeasurementValid
    centerTaskValid
    safetyValid
    ekfValid
    zoomControllerValid
    controllerEnable
    jConditionMetric
];

% 检查输入是否包含NaN或Inf。
if any(~isfinite(statusInputs))
    faultCode = 1;
    return;
end

controllerStatus = statusInputs;

% Stage 1只要求左相机中心控制链路有效。
systemReady = double( ...
    inputDataValid > 0.5 && ...
    cameraModelValid > 0.5 && ...
    kinematicsValid > 0.5 && ...
    validLeft > 0.5 && ...
    centerTaskValid > 0.5 && ...
    safetyValid > 0.5 && ...
    controllerEnable > 0.5);

% 按优先级输出主要故障原因。
if inputDataValid <= 0.5
    faultCode = 1;
elseif cameraModelValid <= 0.5
    faultCode = 2;
elseif kinematicsValid <= 0.5
    faultCode = 3;
elseif validLeft <= 0.5
    faultCode = 4;
elseif centerTaskValid <= 0.5
    faultCode = 5;
elseif safetyValid <= 0.5
    faultCode = 6;
elseif controllerEnable <= 0.5
    faultCode = 7;
else
    faultCode = 0;
end
end

== matlab function stereo_ibvs_core/03_Feature_Processing/Normalize and Validate Features ==
  data: visionFeature input; cLMeasured output; cameraIntrinsics input; cRMeasured output; scaleMeasured output; validLeft output; validRight output
function [cLMeasured,cRMeasured,scaleMeasured,validLeft,validRight] = ...
    fcn(visionFeature,cameraIntrinsics)
%#codegen
% 将像素坐标转换为左右相机归一化坐标，并检查输入有效性。
%
% visionFeature:
% [validL; validR; uL; vL; uR; vR; scaleL; scaleR]
%
% cameraIntrinsics:
% [fxL; fyL; cxL; cyL; fxR; fyR; cxR; cyR]

cLMeasured = zeros(2,1);
cRMeasured = zeros(2,1);
scaleMeasured = zeros(2,1);

validLeft = 0;
validRight = 0;

features = reshape(visionFeature,8,1);
intrinsics = reshape(cameraIntrinsics,8,1);

% 非有限数据直接判为无效。
if any(~isfinite(features)) || any(~isfinite(intrinsics))
    return;
end

validLRaw = features(1);
validRRaw = features(2);

uL = features(3);
vL = features(4);
uR = features(5);
vR = features(6);

scaleL = features(7);
scaleR = features(8);

fxL = intrinsics(1);
fyL = intrinsics(2);
cxL = intrinsics(3);
cyL = intrinsics(4);

fxR = intrinsics(5);
fyR = intrinsics(6);
cxR = intrinsics(7);
cyR = intrinsics(8);

epsilon = 1e-9;

leftIntrinsicsValid = ...
    fxL > epsilon && fyL > epsilon;

rightIntrinsicsValid = ...
    fxR > epsilon && fyR > epsilon;

validLeft = double( ...
    validLRaw > 0.5 && ...
    leftIntrinsicsValid && ...
    scaleL > 0);

validRight = double( ...
    validRRaw > 0.5 && ...
    rightIntrinsicsValid && ...
    scaleR > 0);

if validLeft > 0.5
    cLMeasured = [
        (uL - cxL) / fxL
        (vL - cyL) / fyL
    ];

    scaleMeasured(1) = scaleL;
end

if validRight > 0.5
    cRMeasured = [
        (uR - cxR) / fxR
        (vR - cyR) / fyR
    ];

    scaleMeasured(2) = scaleR;
end

% 最终有限值保护。
if any(~isfinite(cLMeasured))
    cLMeasured = zeros(2,1);
    scaleMeasured(1) = 0;
    validLeft = 0;
end

if any(~isfinite(cRMeasured))
    cRMeasured = zeros(2,1);
    scaleMeasured(2) = 0;
    validRight = 0;
end
end

== matlab function stereo_ibvs_core/04_FR3_Camera_Kinematics/Express Jacobian in Left Camera ==
  data: Jraw input; JL output; T_CL2B input; valid output
function [JL, valid] = fcn(Jraw, T_CL2B)
%#codegen
% Jraw order from Robotics System Toolbox:
% [angular velocity; linear velocity], expressed in base frame.
%
% JL order used by the controller:
% [linear velocity; angular velocity], expressed in left camera frame.

JL = zeros(6,7);
valid = 0;

if any(~isfinite(Jraw(:))) || any(~isfinite(T_CL2B(:)))
    return;
end

if ~isequal(size(Jraw), [6,7]) || ~isequal(size(T_CL2B), [4,4])
    return;
end

R_B_CL = T_CL2B(1:3,1:3);

rotationError = norm(R_B_CL.' * R_B_CL - eye(3), 'fro');

if rotationError > 1e-5 || abs(det(R_B_CL) - 1) > 1e-5
    return;
end

R_CL_B = R_B_CL.';

Jw_B = Jraw(1:3,:);
Jv_B = Jraw(4:6,:);

Jv_CL = R_CL_B * Jv_B;
Jw_CL = R_CL_B * Jw_B;

JL = [
    Jv_CL
    Jw_CL
];

if all(isfinite(JL(:)))
    valid = 1;
else
    JL = zeros(6,7);
end
end

== matlab function stereo_ibvs_core/02_Camera_Model/Zoom Position to Camera Intrinsics ==
  data: zoomPositionSteps input; cameraIntrinsics output; intrinsicsFixed input; focalLengthPx output; cameraModelValid output
function [cameraIntrinsics,focalLengthPx,cameraModelValid] = ...
    fcn(zoomPositionSteps,intrinsicsFixed)
%#codegen
% 代码作用：
% Stage 1暂时不根据步进电机位置改变相机内参。
% 本函数检查输入是否合法，并输出左右相机的固定内参。
% Stage 5加入变焦后，再将这里替换为“电机步数到相机内参”的标定模型。

% 输入参数含义：
% zoomPositionSteps：
% 左右变焦步进电机的累计位置，格式为：
% [leftSteps; rightSteps]
%
% intrinsicsFixed：
% Stage 1使用的固定相机内参，格式为：
% [fxL; fyL; cxL; cyL; fxR; fyR; cxR; cyR]

% 输出参数含义：
% cameraIntrinsics：
% 左右相机当前使用的内参，格式为：
% [fxL; fyL; cxL; cyL; fxR; fyR; cxR; cyR]
%
% focalLengthPx：
% 左右相机水平方向焦距，单位为像素，格式为：
% [fxL; fxR]
%
% cameraModelValid：
% 相机模型是否有效。有效为1，无效为0。

cameraIntrinsics = zeros(8,1);
focalLengthPx = zeros(2,1);
cameraModelValid = 0;

steps = reshape(zoomPositionSteps,2,1);
intrinsics = reshape(intrinsicsFixed,8,1);

% 检查输入中是否存在NaN或Inf。
if any(~isfinite(steps)) || any(~isfinite(intrinsics))
    return;
end

fxL = intrinsics(1);
fyL = intrinsics(2);
fxR = intrinsics(5);
fyR = intrinsics(6);

% 焦距必须为正数。
if fxL <= 0 || fyL <= 0 || fxR <= 0 || fyR <= 0
    return;
end

% Stage 1直接采用固定内参。
cameraIntrinsics = intrinsics;
focalLengthPx = [fxL; fxR];
cameraModelValid = 1;
end

== matlab function stereo_ibvs_core/07_Arm_Priority_Controller/Stage1 Center Task Controller ==
  data: cLMeasured input; qDotCenter output; JL input; validLeft input; cameraModelValid input; kinematicsValid input; controllerEnable input; centerDesired input; rhoStage1 input; Kc input; lambdaC input; centerError output; centerTaskValid output; jConditionMetric output
function [qDotCenter,centerError,centerTaskValid,jConditionMetric] = ...
    fcn(cLMeasured,JL,validLeft,cameraModelValid,kinematicsValid, ...
    controllerEnable,centerDesired,rhoStage1,Kc,lambdaC)
%#codegen
% 代码作用：
% 根据左相机归一化中心误差计算Stage 1关节速度。
% 当前使用固定逆深度，不包含目标速度前馈、深度次任务和零空间任务。

% 输入参数含义：
% cLMeasured：
% 左相机目标归一化坐标，[xL; yL]。
%
% JL：
% 左相机光心雅可比，尺寸为6×7。
% 速度排列为[线速度; 角速度]，并在左相机坐标系表达。
%
% validLeft：
% 左相机目标是否有效。
%
% cameraModelValid：
% 当前相机内参模型是否有效。
%
% kinematicsValid：
% 当前机械臂运动学计算是否有效。
%
% controllerEnable：
% 控制器总使能信号。
%
% centerDesired：
% 期望归一化中心坐标，通常为[0;0]。
%
% rhoStage1：
% Stage 1使用的固定逆深度，rho=1/Z。
%
% Kc：
% 左相机中心任务反馈增益，尺寸为2×2。
%
% lambdaC：
% 中心任务阻尼伪逆系数。

% 输出参数含义：
% qDotCenter：
% 左相机中心任务产生的7维关节速度，单位rad/s。
%
% centerError：
% 当前归一化中心误差。
%
% centerTaskValid：
% 本次中心任务计算是否有效，有效为1，无效为0。
%
% jConditionMetric：
% 中心任务雅可比的条件指标。
% 数值越接近0，说明当前任务越接近奇异状态。

qDotCenter = zeros(7,1);
centerError = zeros(2,1);
centerTaskValid = 0;
jConditionMetric = 0;

cL = reshape(cLMeasured,2,1);
cLd = reshape(centerDesired,2,1);
JLeft = reshape(JL,6,7);
gainC = reshape(Kc,2,2);

% 检查所有输入是否为有限值。
if any(~isfinite(cL)) || ...
        any(~isfinite(cLd)) || ...
        any(~isfinite(JLeft(:))) || ...
        any(~isfinite(gainC(:))) || ...
        ~isfinite(rhoStage1) || ...
        ~isfinite(lambdaC)
    return;
end

% 检查控制器及相关输入是否有效。
if validLeft <= 0.5 || ...
        cameraModelValid <= 0.5 || ...
        kinematicsValid <= 0.5 || ...
        controllerEnable <= 0.5
    return;
end

if rhoStage1 <= 0 || lambdaC < 0
    return;
end

xL = cL(1);
yL = cL(2);
rho = rhoStage1;

centerError = cL - cLd;

% 左相机归一化点特征交互矩阵。
Lc = [
    -rho, 0, xL*rho, xL*yL, -(1+xL*xL), yL
    0, -rho, yL*rho, 1+yL*yL, -xL*yL, -xL
];

% 将相机速度任务映射到7维关节空间。
Jc = Lc * JLeft;

% Stage 1暂时不使用目标运动前馈。
nuC = -gainC * centerError;

% 阻尼最小二乘矩阵。
G = Jc * Jc.' + lambdaC^2 * eye(2);

% 计算简单的条件指标。
detG = G(1,1)*G(2,2) - G(1,2)*G(2,1);
traceG = G(1,1) + G(2,2);

jConditionMetric = detG / ...
    (traceG*traceG + 1e-12);

if detG <= 0 || any(~isfinite(G(:)))
    return;
end

% 阻尼伪逆：
% qDot = Jc' * inv(Jc*Jc' + lambda^2*I) * nuC
qDotCenter = Jc.' * (G \ nuC);

if any(~isfinite(qDotCenter))
    qDotCenter = zeros(7,1);
    return;
end

centerTaskValid = 1;
end

== matlab function stereo_ibvs_core/09_Safety_Supervisor/MATLAB Function ==
  data: qDotRaw input; qDotSafe output; q input; centerTaskValid input; controllerEnable input; cameraMountCalibrated input; qMin input; qMax input; qLimitSoftMargin input; qDotMax input; jointLimitWarning output; velocitySaturationFlag output; safetyValid output
function [qDotSafe,jointLimitWarning,velocitySaturationFlag,safetyValid] = ...
    fcn(qDotRaw,q,centerTaskValid,controllerEnable,cameraMountCalibrated, ...
    qMin,qMax,qLimitSoftMargin,qDotMax)
%#codegen
% 代码作用：
% 对控制器产生的7维关节速度进行有限值检查、速度限幅和关节软限位保护。
% 当输入无效、控制器未使能或手眼标定未完成时，输出零关节速度。

% 输入参数含义：
% qDotRaw：
% 控制器计算出的原始7维关节速度，单位rad/s。
%
% q：
% 当前FR3的7维关节位置，单位rad。
%
% centerTaskValid：
% 中心任务本次计算是否有效。
%
% controllerEnable：
% 控制器总使能信号。
%
% cameraMountCalibrated：
% 左相机与fr3_link8之间的手眼安装矩阵是否已经完成标定。
%
% qMin、qMax：
% FR3七个关节的最小和最大允许位置，单位rad。
%
% qLimitSoftMargin：
% 关节软限位保护距离，单位rad。
%
% qDotMax：
% Simulink算法层允许的最大关节速度，单位rad/s。

% 输出参数含义：
% qDotSafe：
% 经过安全检查后的7维关节速度，单位rad/s。
%
% jointLimitWarning：
% 每个关节是否进入软限位区域，进入为1，否则为0。
%
% velocitySaturationFlag：
% 每个关节是否发生速度限幅，发生为1，否则为0。
%
% safetyValid：
% 当前是否允许输出非零关节速度，允许为1，否则为0。

qDotSafe = zeros(7,1);
jointLimitWarning = zeros(7,1);
velocitySaturationFlag = zeros(7,1);
safetyValid = 0;

qDotCandidate = reshape(qDotRaw,7,1);
qCurrent = reshape(q,7,1);
qLower = reshape(qMin,7,1);
qUpper = reshape(qMax,7,1);
qDotLimit = reshape(qDotMax,7,1);

% 检查输入是否包含NaN或Inf。
if any(~isfinite(qDotCandidate)) || ...
        any(~isfinite(qCurrent)) || ...
        any(~isfinite(qLower)) || ...
        any(~isfinite(qUpper)) || ...
        any(~isfinite(qDotLimit)) || ...
        ~isfinite(qLimitSoftMargin)
    return;
end

% 检查控制链路是否允许输出速度。
if centerTaskValid <= 0.5 || ...
        controllerEnable <= 0.5 || ...
        cameraMountCalibrated <= 0.5
    return;
end

if qLimitSoftMargin <= 0 || ...
        any(qUpper <= qLower) || ...
        any(qDotLimit <= 0)
    return;
end

% 关节速度逐元素限幅。
qDotLimited = min(max(qDotCandidate,-qDotLimit),qDotLimit);

velocitySaturationFlag = double( ...
    abs(qDotLimited-qDotCandidate) > 1e-12);

% 关节软限位保护。
for i = 1:7
    nearLowerLimit = ...
        qCurrent(i)-qLower(i) <= qLimitSoftMargin;

    nearUpperLimit = ...
        qUpper(i)-qCurrent(i) <= qLimitSoftMargin;

    jointLimitWarning(i) = double( ...
        nearLowerLimit || nearUpperLimit);

    % 接近下限时，禁止继续向下限方向运动。
    if nearLowerLimit && qDotLimited(i) < 0
        qDotLimited(i) = 0;
    end

    % 接近上限时，禁止继续向上限方向运动。
    if nearUpperLimit && qDotLimited(i) > 0
        qDotLimited(i) = 0;
    end

    % 已经越过硬限位时，同样禁止继续向外运动。
    if qCurrent(i) <= qLower(i) && qDotLimited(i) < 0
        qDotLimited(i) = 0;
    end

    if qCurrent(i) >= qUpper(i) && qDotLimited(i) > 0
        qDotLimited(i) = 0;
    end
end

if any(~isfinite(qDotLimited))
    return;
end

qDotSafe = qDotLimited;
safetyValid = 1;
end

== matlab function stereo_ibvs_core/01_Input_Validity/MATLAB Function ==
  data: qRaw input; q output; visionFeatureRaw input; zoomPositionStepsRaw input; controllerEnableRaw input; resetRaw input; qInitial input; zoomInitialSteps input; visionFeature output; zoomPositionSteps output; controllerEnableSafe output; resetSafe output; inputDataValid output
function [q,visionFeature,zoomPositionSteps,controllerEnableSafe, ...
    resetSafe,inputDataValid] = ...
    fcn(qRaw,visionFeatureRaw,zoomPositionStepsRaw, ...
    controllerEnableRaw,resetRaw,qInitial,zoomInitialSteps)
%#codegen
% 代码作用：
% 检查模型顶层输入是否包含NaN或Inf。
% 合法输入会被保存；非法输入使用最近一次合法值代替，
% 同时关闭控制器，防止无效数据进入运动学和控制模块。

% 输入参数含义：
% qRaw：
% ROS或仿真输入的FR3七维关节位置，单位rad。
%
% visionFeatureRaw：
% 双目视觉特征，格式为：
% [validL; validR; uL; vL; uR; vR; scaleL; scaleR]
%
% zoomPositionStepsRaw：
% 左右变焦步进电机累计位置：
% [leftSteps; rightSteps]
%
% controllerEnableRaw：
% 外部控制器使能信号。
%
% resetRaw：
% 控制器和估计器复位信号。
%
% qInitial：
% 输入无效时使用的初始安全关节位置。
%
% zoomInitialSteps：
% 输入无效时使用的初始变焦电机位置。

% 输出参数含义：
% q：
% 检查后的七维关节位置。
%
% visionFeature：
% 检查后的双目视觉特征。
%
% zoomPositionSteps：
% 检查后的左右变焦电机累计位置。
%
% controllerEnableSafe：
% 安全控制使能。只有全部输入有效时才允许为1。
%
% resetSafe：
% 检查后的复位信号。
%
% inputDataValid：
% 本周期全部输入是否有效，有效为1，无效为0。

persistent lastQ
persistent lastVisionFeature
persistent lastZoomPositionSteps

initialQ = reshape(qInitial,7,1);
initialZoom = reshape(zoomInitialSteps,2,1);

if isempty(lastQ)
    lastQ = initialQ;
    lastVisionFeature = zeros(8,1);
    lastZoomPositionSteps = initialZoom;
end

qCandidate = reshape(qRaw,7,1);
visionCandidate = reshape(visionFeatureRaw,8,1);
zoomCandidate = reshape(zoomPositionStepsRaw,2,1);

qValid = all(isfinite(qCandidate));
visionValid = all(isfinite(visionCandidate));
zoomValid = all(isfinite(zoomCandidate));
enableValid = isfinite(controllerEnableRaw);
resetValid = isfinite(resetRaw);

if qValid
    lastQ = qCandidate;
end

if visionValid
    lastVisionFeature = visionCandidate;
end

if zoomValid
    lastZoomPositionSteps = zoomCandidate;
end

q = lastQ;
visionFeature = lastVisionFeature;
zoomPositionSteps = lastZoomPositionSteps;

inputDataValid = double( ...
    qValid && ...
    visionValid && ...
    zoomValid && ...
    enableValid && ...
    resetValid);

controllerEnableSafe = double( ...
    inputDataValid > 0.5 && ...
    controllerEnableRaw > 0.5);

if resetValid
    resetSafe = double(resetRaw > 0.5);
else
    resetSafe = 0;
end

% 复位时清除历史输入。
if resetSafe > 0.5
    lastQ = initialQ;
    lastVisionFeature = zeros(8,1);
    lastZoomPositionSteps = initialZoom;

    q = lastQ;
    visionFeature = lastVisionFeature;
    zoomPositionSteps = lastZoomPositionSteps;
    controllerEnableSafe = 0;
end
end
